simulink model "FuelPumpControlModel"  (R2024a)
settings: Solver=VariableStepAuto  StartTime=0.0  StopTime=10  RelTol=1e-3
settings Model: Creator=ec97883  LastModifiedBy=ec97883

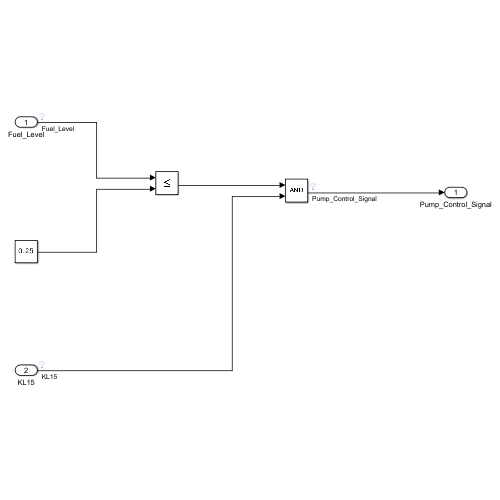
[thumbnail: Simulink's stored preview of the top-level diagram]
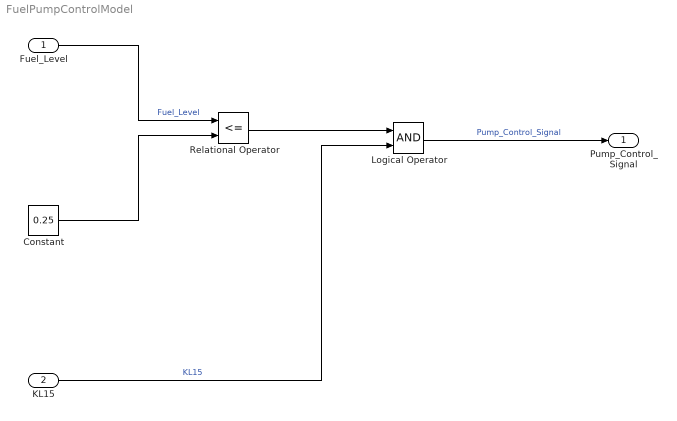
== system FuelPumpControlModel ==
  Fuel_Level : Inport  OutDataTypeStr=double
  KL15 : Inport  Port=2  OutDataTypeStr=boolean  PortDimensions=1
  Constant : Constant  Value=0.25  OutDataTypeStr=double
  Logical Operator : Logic  AllPortsSameDT=off  OutDataTypeStr=boolean
  Relational Operator : RelationalOperator  Operator=<=  OutDataTypeStr=boolean  RndMeth=Simplest  InputSameDT=off
  Pump_Control_Signal : Outport  OutDataTypeStr=boolean  PortDimensions=1
  wires:
  Fuel_Level/1 -> Relational Operator/1  "Fuel_Level"
  Constant/1 -> Relational Operator/2
  Relational Operator/1 -> Logical Operator/1
  KL15/1 -> Logical Operator/2  "KL15"
  Logical Operator/1 -> Pump_Control_Signal/1  "Pump_Control_Signal"
